simulink model "test_accurateTiltingModel"  (R2022b)
settings: Solver=ode4  StartTime=0.0  StopTime=20  FixedStep=0.0001  RelTol=1e-3
undefined symbols (not defined in the file): alpha_0, beta, c_direction, I_b, I_i, k_m, k_t, m_b, N, p_mot, w_bar_0, x_0
libraries: uavutilslib x2
settings Model: PacingRate=0.100000  Creator=pozzan  LastModifiedBy=pozzan

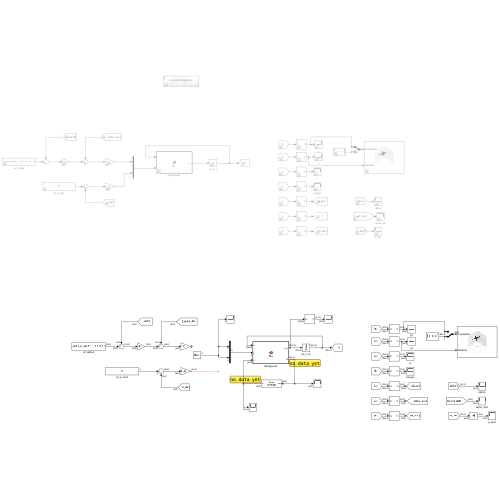
[thumbnail: Simulink's stored preview of the top-level diagram]
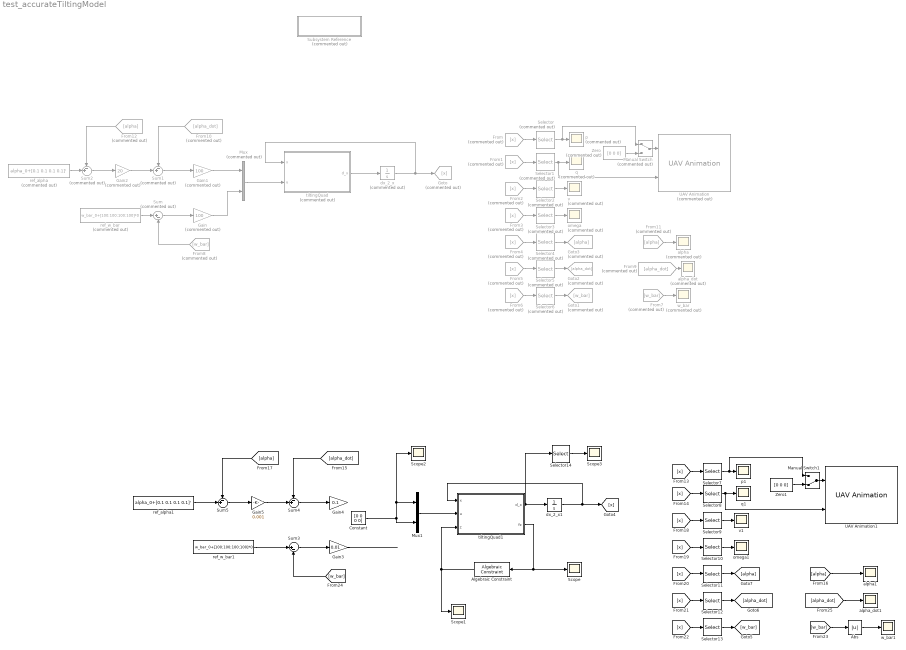
== system test_accurateTiltingModel ==
  Abs : Abs  SaturateOnIntegerOverflow=off
  Algebraic Constraint : AlgebraicConstraint  InitialGuess=zeros(N,1)
  Constant : Constant  Value=[0 0 0 0]
  From{,1..6} (7 alike) : From  Commented=on  GotoTag=x
  From10 : From  Commented=on  GotoTag=alpha_dot
  From11 : From  Commented=on  GotoTag=alpha
  From12 : From  Commented=on  GotoTag=alpha
  From7 : From  Commented=on  GotoTag=w_bar
  From8 : From  Commented=on  GotoTag=w_bar
  From9 : From  Commented=on  GotoTag=alpha_dot
  Gain : Gain  Commented=on  Gain=100
  Gain1 : Gain  Commented=on  Gain=100
  Gain2 : Gain  Commented=on  Gain=20
  Gain3 : Gain  Gain=0.01
  Gain4 : Gain  Gain=0.1
  Gain5 : Gain  Gain=0.001
  Goto : Goto  Commented=on  GotoTag=x
  Goto1 : Goto  Commented=on  GotoTag=w_bar
  Goto2 : Goto  Commented=on  GotoTag=alpha_dot
  Goto3 : Goto  Commented=on  GotoTag=alpha
  Manual Switch : ManualSwitch  Commented=on
  Manual Switch1 : ManualSwitch  CurrentSetting=0
  Mux : Mux  Commented=on  Inputs=2
  Mux1 : Mux  Inputs=2
  Scope{,1..3} (4 alike) : Scope
  Selector : Selector  Commented=on  InputPortWidth=25  IndexOptions=Index vector (dialog)  Indices=1:3  OutputSizes=1
  Selector1 : Selector  Commented=on  InputPortWidth=25  IndexOptions=Index vector (dialog)  Indices=4:7  OutputSizes=1
  Selector10 : Selector  InputPortWidth=13+3*N  IndexOptions=Index vector (dialog)  Indices=11:13  OutputSizes=1
  Selector11 : Selector  InputPortWidth=13+3*N  IndexOptions=Index vector (dialog)  Indices=14:14+N-1  OutputSizes=1
  Selector12 : Selector  InputPortWidth=13+3*N  IndexOptions=Index vector (dialog)  Indices=14+N:14+2*N-1  OutputSizes=1
  Selector13 : Selector  InputPortWidth=13+3*N  IndexOptions=Index vector (dialog)  Indices=14+2*N:14+3*N-1  OutputSizes=1
  Selector14 : Selector  InputPortWidth=13+3*N  IndexOptions=Index vector (dialog)  Indices=14+N:14+2*N-1  OutputSizes=1
  Selector2 : Selector  Commented=on  InputPortWidth=25  IndexOptions=Index vector (dialog)  Indices=8:10  OutputSizes=1
  Selector3 : Selector  Commented=on  InputPortWidth=25  IndexOptions=Index vector (dialog)  Indices=11:13  OutputSizes=1
  Selector4 : Selector  Commented=on  InputPortWidth=25  IndexOptions=Index vector (dialog)  Indices=14:17  OutputSizes=1
  Selector5 : Selector  Commented=on  InputPortWidth=25  IndexOptions=Index vector (dialog)  Indices=18:21  OutputSizes=1
  Selector6 : Selector  Commented=on  InputPortWidth=25  IndexOptions=Index vector (dialog)  Indices=22:25  OutputSizes=1
  Selector7 : Selector  InputPortWidth=13+3*N  IndexOptions=Index vector (dialog)  Indices=1:3  OutputSizes=1
  Selector8 : Selector  InputPortWidth=13+3*N  IndexOptions=Index vector (dialog)  Indices=4:7  OutputSizes=1
  Selector9 : Selector  InputPortWidth=13+3*N  IndexOptions=Index vector (dialog)  Indices=8:10  OutputSizes=1
  Subsystem Reference : Subsystem  Commented=on  ReferencedSubsystem=accurateTiltingModel
  Sum : Sum  Commented=on  Inputs=|+-
  Sum1 : Sum  Commented=on  Inputs=-+|
  Sum2 : Sum  Commented=on  Inputs=-+|
  Sum3 : Sum  Inputs=|+-
  Sum4 : Sum  Inputs=-+|
  Sum5 : Sum  Inputs=-+|
  UAV Animation : uavutilslib/UAV Animation  Commented=on  UAVType=Multirotor  UAVSize=1  InertialZDirection=Up  SampleTime=0.02
  UAV Animation1 : uavutilslib/UAV Animation  UAVType=Multirotor  UAVSize=1  InertialZDirection=Up  SampleTime=0.02
  Zero : Constant  Commented=on  Value=[0 0 0]  OutDataTypeStr=Inherit: Inherit via back propagation
  Zero1 : Constant  Value=[0 0 0]  OutDataTypeStr=Inherit: Inherit via back propagation
  alpha : Scope  Commented=on
  alpha1 : Scope
  alpha_dot : Scope  Commented=on
  alpha_dot1 : Scope
  dx_2_x : Integrator  Commented=on  InitialCondition=x_0
  dx_2_x1 : Integrator  InitialCondition=x_0
  omega : Scope  Commented=on
  omega1 : Scope
  p : Scope  Commented=on
  p1 : Scope
  q : Scope  Commented=on
  q1 : Scope
  ref_alpha : Constant  Commented=on  Value=alpha_0+[0.1 0.1 0.1 0.1]'  VectorParams1D=off
  ref_alpha1 : Constant  Value=alpha_0+[0.1 0.1 0.1 0.1]'  VectorParams1D=off
  ref_w_bar : Constant  Commented=on  Value=w_bar_0+[100;100;100;100]*0
  ref_w_bar1 : Constant  Value=w_bar_0+[100;100;100;100]*0
  tiltingQuad : MATLAB Function  Commented=on  TreatAsAtomicUnit=on
  tiltingQuad1 : MATLAB Function  TreatAsAtomicUnit=on
  v : Scope  Commented=on
  v1 : Scope
  w_bar : Scope  Commented=on
  w_bar1 : Scope
  wires:
  tiltingQuad/1(d_x) -> dx_2_x/1
  dx_2_x/1 -> Goto/1, tiltingQuad/1(x)
  Mux/1 -> tiltingQuad/2(u)
  From/1 -> Selector/1
  Selector/1 -> Manual Switch/1, p/1
  From1/1 -> Selector1/1
  Selector1/1 -> UAV Animation/2, q/1
  From2/1 -> Selector2/1
  Selector2/1 -> v/1
  From3/1 -> Selector3/1
  Selector3/1 -> omega/1
  From4/1 -> Selector4/1
  Selector4/1 -> Goto3/1
  From5/1 -> Selector5/1
  Selector5/1 -> Goto2/1
  From6/1 -> Selector6/1
  Selector6/1 -> Goto1/1
  From7/1 -> w_bar/1
  Gain1/1 -> Mux/1
  Gain/1 -> Mux/2
  Sum/1 -> Gain/1
  From8/1 -> Sum/2
  ref_w_bar/1 -> Sum/1
  From9/1 -> alpha_dot/1
  Sum1/1 -> Gain1/1
  From10/1 -> Sum1/1
  ref_alpha/1 -> Sum2/2
  From11/1 -> alpha/1
  Gain2/1 -> Sum1/2
  Sum2/1 -> Gain2/1
  From12/1 -> Sum2/1
  Manual Switch/1 -> UAV Animation/1
  Zero/1 -> Manual Switch/2
  [x] -> Selector10/1
  [x] -> Selector9/1
  dx_2_x1/1 -> [x], tiltingQuad1/1(x)
  Sum5/1 -> Gain5/1
  Selector7/1 -> Manual Switch1/1, p1/1
  Selector12/1 -> [alpha_dot]
  Gain5/1 -> Sum4/2
  ref_alpha1/1 -> Sum5/2
  [alpha_dot] -> alpha_dot1/1
  [w_bar] -> Abs/1
  [alpha] -> alpha1/1
  [x] -> Selector7/1
  Selector13/1 -> [w_bar]
  [alpha] -> Sum5/1
  ref_w_bar1/1 -> Sum3/1
  [x] -> Selector8/1
  [alpha_dot] -> Sum4/1
  Sum3/1 -> Gain3/1
  [w_bar] -> Sum3/2
  Constant/1 -> Mux1/2, Scope2/1, Mux1/1
  Gain3/1 -> ?
  Sum4/1 -> Gain4/1
  Manual Switch1/1 -> UAV Animation1/1
  Selector11/1 -> [alpha]
  [x] -> Selector13/1
  Selector10/1 -> omega1/1
  Selector8/1 -> UAV Animation1/2, q1/1
  Zero1/1 -> Manual Switch1/2
  [x] -> Selector11/1
  [x] -> Selector12/1
  Selector9/1 -> v1/1
  tiltingQuad1/2(fz) -> Scope/1, Algebraic Constraint/1
  Algebraic Constraint/1 -> Scope1/1, tiltingQuad1/3(z)
  Mux1/1 -> tiltingQuad1/2(u)
  Abs/1 -> w_bar1/1
  tiltingQuad1/1(d_x) -> Selector14/1, dx_2_x1/1
  Selector14/1 -> Scope3/1

== matlab function test_accurateTiltingModel/tiltingQuad ==
  data: x input; u input; d_x output; m_b parameter; beta parameter; I_b parameter; I_i parameter; c_direction parameter; k_m parameter; k_t parameter; p_mot parameter
function d_x = fcn(x, u, m_b, beta, I_b, I_i, c_direction, k_m, k_t, p_mot)

% state x: [p q v omega alpha alpha_dot w_bar]
% input u: [alpha_ddot w_bar_dot]
% output: dot_x
% parameters
%   m_b: drone mass [kg]
%   beta: propellers tilting plane yaw angle [rad]
%   I_b: main body inertia [Kg*m^2]
%   I_i: rotor+propeller inertia [Kg*m^2]
%   c_direction: propeller tourning direction (1:CCW, -1:CW)
%   k_m: propeller drag coefficient [Nm/s^2]
%   k_t: propeller torque coefficient [Nm/s^2]
%   p_mot: rotor position w.r.t. body


% position of c.o.m. w.r.t. globa frame
p = x(1:3);
% quaternion associated to B2W rotation
q = x(4:7);
% linear velocity of c.o.m. expressed in world frame
v = x(8:10);
% angular velocity expressed in body frame
omega = x(11:13);
% tilting angles
alpha = x(14:17);
% tilting angle rates
alpha_dot = x(18:21);
% spinning rate
w_bar = x(22:25);

% tilting angle accelerations
alpha_ddot = u(1:4);
% spinning rate accelerations
w_bar_dot = u(5:8);

% output vector initialization
d_x = zeros(size(x));

% body to world quaternion manipulation
eta = q(1);
epsilon = q(2:4);
epsilon_x = [0, -epsilon(3), epsilon(2); epsilon(3), 0, -epsilon(1); -epsilon(2), epsilon(1), 0]; 
Rq = eye(3) + 2*eta*epsilon_x + 2*epsilon_x^2;  % rotation matrix, body to world
Mq = [eta, -epsilon'; epsilon, eta*eye(3)+epsilon_x]; % quaternion composition matrix
% quaternion derivative
d_q = 1/2*Mq*[0;omega];

% total quadrotor inertia
I_tot = I_b;
% dynamics components depending on omegas
B_terms = cross(omega,I_b*omega);
% total body torques (due to thrust)
tau_b = zeros(3,1);
T_b = zeros(3,1);

for k=1:4
    % rotor to body rotation matrix
    B_R_i = axang2rotm([0 0 1 beta(k)])*axang2rotm([1 0 0 alpha(k)]);
    % time derivative of rotor to body rotation matrix
    B_R_i_dot = B_R_i * [0 0 0; 0 0 -alpha_dot(k); 0 alpha_dot(k) 0];
    % angular rate of the i-th rotor in the i-th rotor frame
    omega_i = B_R_i.' * omega + [alpha_dot(k); 0; w_bar(k)];
    
    % drag torque
    tau_ei = [0;0; -k_m*omega_i(3)*abs(omega_i(3))];

    % thrust in body frame
    T_i = B_R_i* [0;0;c_direction(k)*k_t*w_bar(k)*abs(w_bar(k))];
    tau_b = tau_b + cross(p_mot(k,:)',T_i);
    T_b = T_b + T_i;

    % add rotor inetria to total inertia
    I_tot = I_tot + B_R_i*I_i*B_R_i';
    % add rotor B dynamics to total B dyn
    B_terms = B_terms +...
        B_R_i * (...
        I_i*B_R_i_dot.'*omega + I_i*[alpha_ddot(k); 0; w_bar_dot(k)] +...
        cross(omega_i,I_i*omega_i) - tau_ei ...
        );
end

d_v = [0;0;-9.81] + 1/m_b*Rq*T_b;
d_omega = I_tot\(tau_b-B_terms);


%% output filling

d_x(1:3) = v;
d_x(4:7) = d_q;
d_x(8:10) = d_v;
d_x(11:13) = d_omega;
d_x(14:17) = alpha_dot;
d_x(18:21) = alpha_ddot;
d_x(22:25) = w_bar_dot;

== matlab function test_accurateTiltingModel/tiltingQuad1 ==
  data: x input; u input; z input; d_x output; m_b parameter; beta parameter; I_b parameter; I_i parameter; c_direction parameter; k_m parameter; k_t parameter; p_mot parameter; fz output
function [d_x, fz] = fcn(x, u, z, m_b, beta, I_b, I_i, c_direction, k_m, k_t, p_mot)

% state x: [p q v omega alpha alpha_dot w_bar]
% input u: [tau_i_x tau_i_z]
% input z: algebraic state: tau_i_y
% output:
%   dot_x
%   fz: algebraic state
% parameters
%   m_b: drone mass [kg]
%   beta: propellers tilting plane yaw angle [rad]
%   I_b: main body inertia [Kg*m^2]
%   I_i: rotor+propeller inertia [Kg*m^2]
%   c_direction: propeller tourning direction (1:CCW, -1:CW)
%   k_m: propeller drag coefficient [Nm/s^2]
%   k_t: propeller torque coefficient [Nm/s^2]
%   p_mot: rotor position w.r.t. body

N = 4;
p_ind = 1:3;
q_ind = 4:7;
v_ind = 8:10;
omega_ind = 11:13;
alpha_ind = 14:14+N-1;
alpha_dot_ind = 14+N:14+2*N-1;
w_bar_ind = 14+2*N:14+3*N-1;

tau_i_x_ind = 1:N;
tau_i_z_ind = N+1:2*N;



% position of c.o.m. w.r.t. globa frame
p = x(p_ind);
% quaternion associated to B2W rotation
q = x(q_ind);
% linear velocity of c.o.m. expressed in world frame
v = x(v_ind);
% angular velocity expressed in body frame
omega = x(omega_ind);
% tilting angles
alpha = x(alpha_ind);
% tilting angle rates
alpha_dot = x(alpha_dot_ind);
% spinning rate
w_bar = x(w_bar_ind);

% tilting angle accelerations
tau_i_x = u(tau_i_x_ind);
% spinning rate accelerations
tau_i_z = u(tau_i_z_ind);

% output vector initialization
d_x = zeros(size(x));
fz = zeros(size(z));
alpha_ddot = zeros(size(alpha));
w_bar_dot = zeros(size(w_bar));

% propeller torques composition
tau_i = [
    tau_i_x.'
    z.'
    tau_i_z.'
    ];

% body to world quaternion manipulation
eta = q(1);
epsilon = q(2:4);
epsilon_x = [0, -epsilon(3), epsilon(2); epsilon(3), 0, -epsilon(1); -epsilon(2), epsilon(1), 0]; 
Rq = eye(3) + 2*eta*epsilon_x + 2*epsilon_x^2;  % rotation matrix, body to world
Mq = [eta, -epsilon'; epsilon, eta*eye(3)+epsilon_x]; % quaternion composition matrix
% quaternion derivative
d_q = 1/2*Mq*[0;omega];

% coriolis componentes of the body
coriol_b = cross(omega,I_b*omega);
% total body thrust
T_b = zeros(3,1);
% total body torque (due to thrust)
tau_b = zeros(3,1);
% total propellers torque in body frame
b_tau_i = zeros(3,1);

for k=1:N
    % rotor to body rotation matrix
    B_R_i = axang2rotm([0 0 1 beta(k)])*axang2rotm([1 0 0 alpha(k)]);

    % thrust of i-th prop in **body** frame
    T_i = B_R_i* [0;0;c_direction(k)*k_t*w_bar(k)*abs(w_bar(k))];
    % update total torque in body frame
    tau_b = tau_b + cross(p_mot(k,:)',T_i);
    % update total thrust in body frame
    T_b = T_b + T_i;
    % update propellers torque in body frame
    b_tau_i = b_tau_i + B_R_i*tau_i(:,k);

    
end

d_v = [0;0;-9.81] + 1/m_b*Rq*T_b;
d_omega = I_b\(tau_b-coriol_b-b_tau_i);

for k=1:N
    % rotor to body rotation matrix
    B_R_i = axang2rotm([0 0 1 beta(k)])*axang2rotm([1 0 0 alpha(k)]);
    % time derivative of rotor to body rotation matrix
    B_R_i_dot = B_R_i * [0 0 0; 0 0 -alpha_dot(k); 0 alpha_dot(k) 0];
    % angular rate of the i-th rotor in the i-th rotor frame
    omega_i = B_R_i.' * omega + [alpha_dot(k); 0; w_bar(k)];
    
    % drag torque
    tau_ei = [0;0; -k_m*omega_i(3)*abs(omega_i(3))];
    
    % [ddot_alpha_1; 0; dot_w_bar_i]
    d_omega_rel = I_i\(tau_i(:,k)+tau_ei-cross(omega_i,I_i*omega_i)) - ...
        B_R_i.'*d_omega - B_R_i_dot.'*omega;

    alpha_ddot(k) = d_omega_rel(1);
    fz(k) = d_omega_rel(2);
    w_bar_dot(k) = d_omega_rel(3);
end


%% output filling

d_x(p_ind) = v;
d_x(q_ind) = d_q;
d_x(v_ind) = d_v;
d_x(omega_ind) = d_omega;
d_x(alpha_ind) = alpha_dot;
d_x(alpha_dot_ind) = alpha_ddot;
d_x(w_bar_ind) = w_bar_dot;
